simulink model "c00001M_harness"  (R2018a)
settings: Solver=FixedStepAuto  StartTime=0.0  StopTime=300  FixedStep=0.1  RelTol=1e-3
undefined symbols (not defined in the file): A1, hmax, R1, R2, sigbuilder_block, TempThreshold
(part 1 of 7)
settings Model: Creator=aarrieta  LastModifiedBy=umarkiegi

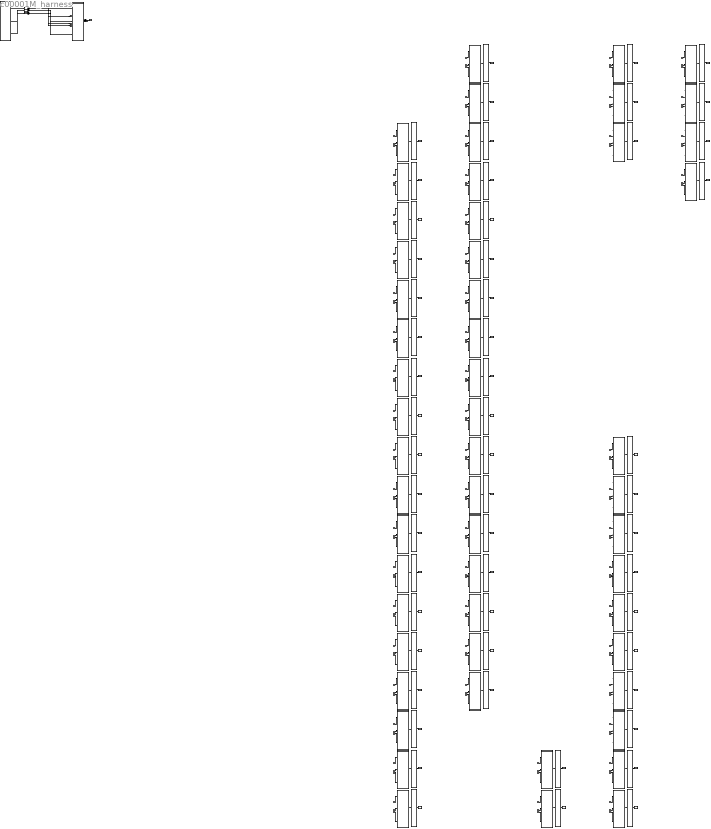
== system c00001M_harness ==
  CPSUT : Subsystem
  Eval100 : Subsystem
  Eval101 : Subsystem
  Eval102 : Subsystem
  Eval103 : Subsystem
  Eval104 : Subsystem
  Eval105 : Subsystem
  Eval106 : Subsystem
  Eval107 : Subsystem
  Eval108 : Subsystem
  Eval109 : Subsystem
  Eval110 : Subsystem
  Eval111 : Subsystem
  Eval112 : Subsystem
  Eval113 : Subsystem
  Eval114 : Subsystem
  Eval115 : Subsystem
  Eval116 : Subsystem
  Eval138 : Subsystem
  Eval139 : Subsystem
  Eval140 : Subsystem
  Eval141 : Subsystem
  Eval142 : Subsystem
  Eval150 : Subsystem
  Eval151 : Subsystem
  Eval152 : Subsystem
  Eval153 : Subsystem
  Eval154 : Subsystem
  Eval155 : Subsystem
  Eval156 : Subsystem
  Eval157 : Subsystem
  Eval158 : Subsystem
  Eval159 : Subsystem
  Eval160 : Subsystem
  Eval161 : Subsystem
  Eval162 : Subsystem
  Eval163 : Subsystem
  Eval82 : Subsystem
  Eval83 : Subsystem
  Eval84 : Subsystem
  Eval85 : Subsystem
  Eval86 : Subsystem
  Eval87 : Subsystem
  Eval88 : Subsystem
  Eval89 : Subsystem
  Eval90 : Subsystem
  Eval91 : Subsystem
  Eval92 : Subsystem
  Eval93 : Subsystem
  Eval94 : Subsystem
  Eval95 : Subsystem
  Eval96 : Subsystem
  Eval97 : Subsystem
  Eval98 : Subsystem
  Eval99 : Subsystem
  Inputs : Subsystem  Tag=STV Subsys  LoadFcn=sigbuilder_block('load');  StartFcn=sigbuilder_block('start');  StopFcn=sigbuilder_block('stop');  ClipboardFcn=sigbuilder_block('clipboard');  mask(Sigbuilder block){tuvar=[0:10]}
      mask init:
      | if ~strcmp(get_param(bdroot(gcb),'SimulationStatus'),'stopped'),tuvar = sigbuilder_block('maskInit'); end
      settings: CopyFcn=sigbuilder_block('copy');  DeleteFcn=sigbuilder_block('delete');  ModelCloseFcn=sigbuilder_block('modelClose');  PreSaveFcn=sigbuilder_block('preSave');  PauseFcn=sigbuilder_block('pause');  ContinueFcn=sigbuilder_block('continue');  NameChangeFcn=sigbuilder_block('namechange');  OpenFcn=sigbuilder_block('open',[276.75 163.5 675.75 486.75 ]);  CloseFcn=sigbuilder_block('close');
      mask Display: plot(0, 0, 100, 100,[2, 2, 32, 32, 2], [68, 8, 8, 68, 68],[32, 2], [38, 38], [32, 19, 2],[53, 60, 44], [32, 17, 17, 2],[16, 16, 31, 31]);txt = getActiveGroup(gcbh);text(2, 100, txt,'verticalAlignment', 'top');
  M083 : Subsystem
  M084 : Subsystem
  M085 : Subsystem
  M086 : Subsystem
  M087 : Subsystem
  M088 : Subsystem
  M089 : Subsystem
  M090 : Subsystem
  M091 : Subsystem
  M092 : Subsystem
  M093 : Subsystem
  M094 : Subsystem
  M095 : Subsystem
  M096 : Subsystem
  M097 : Subsystem
  M098 : Subsystem
  M099 : Subsystem
  M100 : Subsystem
  M101 : Subsystem
  M102 : Subsystem
  M103 : Subsystem
  M104 : Subsystem
  M105 : Subsystem
  M106 : Subsystem
  M107 : Subsystem
  M108 : Subsystem
  M109 : Subsystem
  M110 : Subsystem
  M111 : Subsystem
  M112 : Subsystem
  M113 : Subsystem
  M114 : Subsystem
  M115 : Subsystem
  M116 : Subsystem
  M117 : Subsystem
  M139 : Subsystem
  M140 : Subsystem
  M141 : Subsystem
  M142 : Subsystem
  M143 : Subsystem
  M151 : Subsystem
  M152 : Subsystem
  M153 : Subsystem
  M154 : Subsystem
  M155 : Subsystem
  M156 : Subsystem
  M157 : Subsystem
  M158 : Subsystem
  M159 : Subsystem
  M160 : Subsystem
  M161 : Subsystem
  M162 : Subsystem
  M163 : Subsystem
  M164 : Subsystem
  To Workspace100 : ToWorkspace  VariableName=mutant101  SampleTime=-1
  To Workspace101 : ToWorkspace  VariableName=mutant102  SampleTime=-1
  To Workspace102 : ToWorkspace  VariableName=mutant103  SampleTime=-1
  To Workspace103 : ToWorkspace  VariableName=mutant104  SampleTime=-1
  To Workspace104 : ToWorkspace  VariableName=mutant105  SampleTime=-1
  To Workspace105 : ToWorkspace  VariableName=mutant106  SampleTime=-1
  To Workspace106 : ToWorkspace  VariableName=mutant107  SampleTime=-1
  To Workspace107 : ToWorkspace  VariableName=mutant108  SampleTime=-1
  To Workspace108 : ToWorkspace  VariableName=mutant109  SampleTime=-1
  To Workspace109 : ToWorkspace  VariableName=mutant110  SampleTime=-1
  To Workspace110 : ToWorkspace  VariableName=mutant111  SampleTime=-1
  To Workspace111 : ToWorkspace  VariableName=mutant112  SampleTime=-1
  To Workspace112 : ToWorkspace  VariableName=mutant113  SampleTime=-1
  To Workspace113 : ToWorkspace  VariableName=mutant114  SampleTime=-1
  To Workspace114 : ToWorkspace  VariableName=mutant115  SampleTime=-1
  To Workspace115 : ToWorkspace  VariableName=mutant116  SampleTime=-1
  To Workspace116 : ToWorkspace  VariableName=mutant117  SampleTime=-1
  To Workspace138 : ToWorkspace  VariableName=mutant139  SampleTime=-1
  To Workspace139 : ToWorkspace  VariableName=mutant140  SampleTime=-1
  To Workspace140 : ToWorkspace  VariableName=mutant141  SampleTime=-1
  To Workspace141 : ToWorkspace  VariableName=mutant142  SampleTime=-1
  To Workspace142 : ToWorkspace  VariableName=mutant143  SampleTime=-1
  To Workspace150 : ToWorkspace  VariableName=mutant151  SampleTime=-1
  To Workspace151 : ToWorkspace  VariableName=mutant152  SampleTime=-1
  To Workspace152 : ToWorkspace  VariableName=mutant153  SampleTime=-1
  To Workspace153 : ToWorkspace  VariableName=mutant154  SampleTime=-1
  To Workspace154 : ToWorkspace  VariableName=mutant155  SampleTime=-1
  To Workspace155 : ToWorkspace  VariableName=mutant156  SampleTime=-1
  To Workspace156 : ToWorkspace  VariableName=mutant157  SampleTime=-1
  To Workspace157 : ToWorkspace  VariableName=mutant158  SampleTime=-1
  To Workspace158 : ToWorkspace  VariableName=mutant159  SampleTime=-1
  To Workspace159 : ToWorkspace  VariableName=mutant160  SampleTime=-1
  To Workspace160 : ToWorkspace  VariableName=mutant161  SampleTime=-1
  To Workspace161 : ToWorkspace  VariableName=mutant162  SampleTime=-1
  To Workspace162 : ToWorkspace  VariableName=mutant163  SampleTime=-1
  To Workspace163 : ToWorkspace  VariableName=mutant164  SampleTime=-1
  To Workspace82 : ToWorkspace  VariableName=mutant083  SampleTime=-1
  To Workspace83 : ToWorkspace  VariableName=mutant084  SampleTime=-1
  To Workspace84 : ToWorkspace  VariableName=mutant085  SampleTime=-1
  To Workspace85 : ToWorkspace  VariableName=mutant086  SampleTime=-1
  To Workspace86 : ToWorkspace  VariableName=mutant087  SampleTime=-1
  To Workspace87 : ToWorkspace  VariableName=mutant088  SampleTime=-1
  To Workspace88 : ToWorkspace  VariableName=mutant089  SampleTime=-1
  To Workspace89 : ToWorkspace  VariableName=mutant090  SampleTime=-1
  To Workspace90 : ToWorkspace  VariableName=mutant091  SampleTime=-1
  To Workspace91 : ToWorkspace  VariableName=mutant092  SampleTime=-1
  To Workspace92 : ToWorkspace  VariableName=mutant093  SampleTime=-1
  To Workspace93 : ToWorkspace  VariableName=mutant094  SampleTime=-1
  To Workspace94 : ToWorkspace  VariableName=mutant095  SampleTime=-1
  To Workspace95 : ToWorkspace  VariableName=mutant096  SampleTime=-1
  To Workspace96 : ToWorkspace  VariableName=mutant097  SampleTime=-1
  To Workspace97 : ToWorkspace  VariableName=mutant098  SampleTime=-1
  To Workspace98 : ToWorkspace  VariableName=mutant099  SampleTime=-1
  To Workspace99 : ToWorkspace  VariableName=mutant100  SampleTime=-1
  dtc_CT2 : DataTypeConversion
  dtc_EB2 : DataTypeConversion
  dtc_T2 : DataTypeConversion
  LL2 : Outport
  tag scope: out2=global
  wires:
  CPSUT/1(LL2) -> [out2], LL2/1
  [in7] -> M083/1(CT2)
  [in11] -> M083/2(T2)
  [in12] -> M083/3(EB2)
  M083/1(LL2) -> Eval82/1(In2)
  Eval82/1(Out1) -> To Workspace82/1
  [in7] -> M084/1(CT2)
  [in11] -> M084/2(T2)
  [in12] -> M084/3(EB2)
  M084/1(LL2) -> Eval83/1(In2)
  Eval83/1(Out1) -> To Workspace83/1
  [in7] -> M085/1(CT2)
  [in11] -> M085/2(T2)
  [in12] -> M085/3(EB2)
  M085/1(LL2) -> Eval84/1(In2)
  Eval84/1(Out1) -> To Workspace84/1
  [in7] -> M086/1(CT2)
  [in11] -> M086/2(T2)
  [in12] -> M086/3(EB2)
  M086/1(LL2) -> Eval85/1(In2)
  Eval85/1(Out1) -> To Workspace85/1
  [in7] -> M087/1(CT2)
  [in11] -> M087/2(T2)
  [in12] -> M087/3(EB2)
  M087/1(LL2) -> Eval86/1(In2)
  Eval86/1(Out1) -> To Workspace86/1
  [in7] -> M088/1(CT2)
  [in11] -> M088/2(T2)
  [in12] -> M088/3(EB2)
  M088/1(LL2) -> Eval87/1(In2)
  Eval87/1(Out1) -> To Workspace87/1
  [in7] -> M089/1(CT2)
  [in11] -> M089/2(T2)
  [in12] -> M089/3(EB2)
  M089/1(LL2) -> Eval88/1(In2)
  Eval88/1(Out1) -> To Workspace88/1
  [in7] -> M090/1(CT2)
  [in11] -> M090/2(T2)
  [in12] -> M090/3(EB2)
  M090/1(LL2) -> Eval89/1(In2)
  Eval89/1(Out1) -> To Workspace89/1
  [in7] -> M091/1(CT2)
  [in11] -> M091/2(T2)
  [in12] -> M091/3(EB2)
  M091/1(LL2) -> Eval90/1(In2)
  Eval90/1(Out1) -> To Workspace90/1
  [in7] -> M092/1(CT2)
  [in11] -> M092/2(T2)
  [in12] -> M092/3(EB2)
  M092/1(LL2) -> Eval91/1(In2)
  Eval91/1(Out1) -> To Workspace91/1
  [in7] -> M093/1(CT2)
  [in11] -> M093/2(T2)
  [in12] -> M093/3(EB2)
  M093/1(LL2) -> Eval92/1(In2)
  Eval92/1(Out1) -> To Workspace92/1
  [in7] -> M094/1(CT2)
  [in11] -> M094/2(T2)
  [in12] -> M094/3(EB2)
  M094/1(LL2) -> Eval93/1(In2)
  Eval93/1(Out1) -> To Workspace93/1
  [in7] -> M095/1(CT2)
  [in11] -> M095/2(T2)
  [in12] -> M095/3(EB2)
  M095/1(LL2) -> Eval94/1(In2)
  Eval94/1(Out1) -> To Workspace94/1
  [in7] -> M096/1(CT2)
  [in11] -> M096/2(T2)
  [in12] -> M096/3(EB2)
  M096/1(LL2) -> Eval95/1(In2)
  Eval95/1(Out1) -> To Workspace95/1
  [in7] -> M097/1(CT2)
  [in11] -> M097/2(T2)
  [in12] -> M097/3(EB2)
  M097/1(LL2) -> Eval96/1(In2)
  Eval96/1(Out1) -> To Workspace96/1
  [in7] -> M098/1(CT2)
  [in11] -> M098/2(T2)
  [in12] -> M098/3(EB2)
  M098/1(LL2) -> Eval97/1(In2)
  Eval97/1(Out1) -> To Workspace97/1
  [in7] -> M099/1(CT2)
  [in11] -> M099/2(T2)
  [in12] -> M099/3(EB2)
  M099/1(LL2) -> Eval98/1(In2)
  Eval98/1(Out1) -> To Workspace98/1
  [in7] -> M100/1(CT2)
  [in11] -> M100/2(T2)
  [in12] -> M100/3(EB2)
  M100/1(LL2) -> Eval99/1(In2)
  Eval99/1(Out1) -> To Workspace99/1
  [in7] -> M101/1(CT2)
  [in11] -> M101/2(T2)
  [in12] -> M101/3(EB2)
  M101/1(LL2) -> Eval100/1(In2)
  Eval100/1(Out1) -> To Workspace100/1
  [in7] -> M102/1(CT2)
  [in11] -> M102/2(T2)
  [in12] -> M102/3(EB2)
  M102/1(LL2) -> Eval101/1(In2)
  Eval101/1(Out1) -> To Workspace101/1
  [in7] -> M103/1(CT2)
  [in11] -> M103/2(T2)
  [in12] -> M103/3(EB2)
  M103/1(LL2) -> Eval102/1(In2)
  Eval102/1(Out1) -> To Workspace102/1
  [in7] -> M104/1(CT2)
  [in11] -> M104/2(T2)
  [in12] -> M104/3(EB2)
  M104/1(LL2) -> Eval103/1(In2)
  Eval103/1(Out1) -> To Workspace103/1
  [in7] -> M105/1(CT2)
  [in11] -> M105/2(T2)
  [in12] -> M105/3(EB2)
  M105/1(LL2) -> Eval104/1(In2)
  Eval104/1(Out1) -> To Workspace104/1
  [in7] -> M106/1(CT2)
  [in11] -> M106/2(T2)
  [in12] -> M106/3(EB2)
  M106/1(LL2) -> Eval105/1(In2)
  Eval105/1(Out1) -> To Workspace105/1
  [in7] -> M107/1(CT2)
  [in11] -> M107/2(T2)
  [in12] -> M107/3(EB2)
  M107/1(LL2) -> Eval106/1(In2)
  Eval106/1(Out1) -> To Workspace106/1
  [in7] -> M108/1(CT2)
  [in11] -> M108/2(T2)
  [in12] -> M108/3(EB2)
  M108/1(LL2) -> Eval107/1(In2)
  Eval107/1(Out1) -> To Workspace107/1
  [in7] -> M109/1(CT2)
  [in11] -> M109/2(T2)
  [in12] -> M109/3(EB2)
  M109/1(LL2) -> Eval108/1(In2)
  Eval108/1(Out1) -> To Workspace108/1
  [in7] -> M110/1(CT2)
  [in11] -> M110/2(T2)
  [in12] -> M110/3(EB2)
  M110/1(LL2) -> Eval109/1(In2)
  Eval109/1(Out1) -> To Workspace109/1
  [in7] -> M111/1(CT2)
  [in11] -> M111/2(T2)
  [in12] -> M111/3(EB2)
  M111/1(LL2) -> Eval110/1(In2)
  Eval110/1(Out1) -> To Workspace110/1
  [in7] -> M112/1(CT2)
  [in11] -> M112/2(T2)
  [in12] -> M112/3(EB2)
  M112/1(LL2) -> Eval111/1(In2)
  Eval111/1(Out1) -> To Workspace111/1
  [in7] -> M113/1(CT2)
  [in11] -> M113/2(T2)
  [in12] -> M113/3(EB2)
  M113/1(LL2) -> Eval112/1(In2)
  Eval112/1(Out1) -> To Workspace112/1
  [in7] -> M114/1(CT2)
  [in11] -> M114/2(T2)
  [in12] -> M114/3(EB2)
  M114/1(LL2) -> Eval113/1(In2)
  Eval113/1(Out1) -> To Workspace113/1
  [in7] -> M115/1(CT2)
  [in11] -> M115/2(T2)
  [in12] -> M115/3(EB2)
  M115/1(LL2) -> Eval114/1(In2)
  Eval114/1(Out1) -> To Workspace114/1
  [in7] -> M116/1(CT2)
  [in11] -> M116/2(T2)
  [in12] -> M116/3(EB2)
  M116/1(LL2) -> Eval115/1(In2)
  Eval115/1(Out1) -> To Workspace115/1
  [in7] -> M117/1(CT2)
  [in11] -> M117/2(T2)
  [in12] -> M117/3(EB2)
  M117/1(LL2) -> Eval116/1(In2)
  Eval116/1(Out1) -> To Workspace116/1
  [in7] -> M139/1(CT2)
  [in11] -> M139/2(T2)
  [in12] -> M139/3(EB2)
  M139/1(LL2) -> Eval138/1(In2)
  Eval138/1(Out1) -> To Workspace138/1
  [in7] -> M140/1(CT2)
  [in11] -> M140/2(T2)
  [in12] -> M140/3(EB2)
  M140/1(LL2) -> Eval139/1(In2)
  Eval139/1(Out1) -> To Workspace139/1
  [in7] -> M141/1(CT2)
  [in11] -> M141/2(T2)
  [in12] -> M141/3(EB2)
  M141/1(LL2) -> Eval140/1(In2)
  Eval140/1(Out1) -> To Workspace140/1
  [in7] -> M142/1(CT2)
  [in11] -> M142/2(T2)
  [in12] -> M142/3(EB2)
  M142/1(LL2) -> Eval141/1(In2)
  Eval141/1(Out1) -> To Workspace141/1
  [in7] -> M143/1(CT2)
  [in11] -> M143/2(T2)
  [in12] -> M143/3(EB2)
  M143/1(LL2) -> Eval142/1(In2)
  Eval142/1(Out1) -> To Workspace142/1
  [in7] -> M151/1(CT2)
  [in11] -> M151/2(T2)
  [in12] -> M151/3(EB2)
  M151/1(LL2) -> Eval150/1(In2)
  Eval150/1(Out1) -> To Workspace150/1
  [in7] -> M152/1(CT2)
  [in11] -> M152/2(T2)
  [in12] -> M152/3(EB2)
  M152/1(LL2) -> Eval151/1(In2)
  Eval151/1(Out1) -> To Workspace151/1
  [in7] -> M153/1(CT2)
  [in11] -> M153/2(T2)
  [in12] -> M153/3(EB2)
  M153/1(LL2) -> Eval152/1(In2)
  Eval152/1(Out1) -> To Workspace152/1
  [in7] -> M154/1(CT2)
  [in11] -> M154/2(T2)
  [in12] -> M154/3(EB2)
  M154/1(LL2) -> Eval153/1(In2)
  Eval153/1(Out1) -> To Workspace153/1
  [in7] -> M155/1(CT2)
  [in11] -> M155/2(T2)
  [in12] -> M155/3(EB2)
  M155/1(LL2) -> Eval154/1(In2)
  Eval154/1(Out1) -> To Workspace154/1
  [in7] -> M156/1(CT2)
  [in11] -> M156/2(T2)
  [in12] -> M156/3(EB2)
  M156/1(LL2) -> Eval155/1(In2)
  Eval155/1(Out1) -> To Workspace155/1
  [in7] -> M157/1(CT2)
  [in11] -> M157/2(T2)
  [in12] -> M157/3(EB2)
  M157/1(LL2) -> Eval156/1(In2)
  Eval156/1(Out1) -> To Workspace156/1
  [in7] -> M158/1(CT2)
  [in11] -> M158/2(T2)
  [in12] -> M158/3(EB2)
  M158/1(LL2) -> Eval157/1(In2)
  Eval157/1(Out1) -> To Workspace157/1
  [in7] -> M159/1(CT2)
  [in11] -> M159/2(T2)
  [in12] -> M159/3(EB2)
  M159/1(LL2) -> Eval158/1(In2)
  Eval158/1(Out1) -> To Workspace158/1
  [in7] -> M160/1(CT2)
  [in11] -> M160/2(T2)
  [in12] -> M160/3(EB2)
  M160/1(LL2) -> Eval159/1(In2)
  Eval159/1(Out1) -> To Workspace159/1
  [in7] -> M161/1(CT2)
  [in11] -> M161/2(T2)
  [in12] -> M161/3(EB2)
  M161/1(LL2) -> Eval160/1(In2)
  Eval160/1(Out1) -> To Workspace160/1
  [in7] -> M162/1(CT2)
  [in11] -> M162/2(T2)
  [in12] -> M162/3(EB2)
  M162/1(LL2) -> Eval161/1(In2)
  Eval161/1(Out1) -> To Workspace161/1
  [in7] -> M163/1(CT2)
  [in11] -> M163/2(T2)
  [in12] -> M163/3(EB2)
  M163/1(LL2) -> Eval162/1(In2)
  Eval162/1(Out1) -> To Workspace162/1
  [in7] -> M164/1(CT2)
  [in11] -> M164/2(T2)
  [in12] -> M164/3(EB2)
  M164/1(LL2) -> Eval163/1(In2)
  Eval163/1(Out1) -> To Workspace163/1
  Inputs/1(CT2) -> dtc_CT2/1
  dtc_CT2/1 -> CPSUT/1(CT2), [in7]
  Inputs/2(T2) -> dtc_T2/1
  dtc_T2/1 -> CPSUT/2(T2), [in11]
  Inputs/3(EB2) -> dtc_EB2/1
  dtc_EB2/1 -> CPSUT/3(EB2), [in12]

== system c00001M_harness/CPSUT ==
  note: VALUES
      | ---------------------------------
      | ControlType = 1 | 2 | 3
      | FillTank = 0 | 1
      | EmptyTank = 0 | 1
      | ManualReference between 0 and 1
      | Tempreature between 0 and 100
      | EmergencyButton = 0 | 1
      | LiquidLevel between 0 and 1 (hmax)
  note: Inputs For Tank2
  note: NAMES
      | --------------------------------------------
      | CT1 = ControlType Tank 1
      | F1 = Fill Tank 1
      | E1 = Empty Tank 1
      | MR1 = Manual Reference Tank1
      | T1 = Temperature Tank 1
      | EB1 = Emergency Button Tank 1
      | LL1 = Liquid Level 1
  note: Inputs For Tank3
  note: Inputs For Tank1
  CT2 : Inport
  T2 : Inport  Port=2
  EB2 : Inport  Port=3
  Tank2 : Subsystem
  LL2 : Outport
  wires:
  Tank2/1(LL2) -> LL2/1
  EB2/1 -> Tank2/3(EB2)
  CT2/1 -> Tank2/1(CT2)
  T2/1 -> Tank2/2(T2)

== system c00001M_harness/Eval100 ==
  In2 : Inport
  Constant1 : Constant
  Constant3 : Constant
  Data Type Conversion1 : DataTypeConversion
  Memory2 : Memory  InitialCondition=1
  MinMax : MinMax  Inputs=3
  MinMax2 : MinMax  Inputs=2
  ROOut2 : RelationalOperator  Operator===  OutDataTypeStr=boolean  RndMeth=Simplest
  Out1 : Outport
  wires:
  Data Type Conversion1/1 -> MinMax2/1
  MinMax2/1 -> MinMax/2, Memory2/1
  Memory2/1 -> MinMax2/2
  ROOut2/1 -> Data Type Conversion1/1
  [out2] -> ROOut2/2
  In2/1 -> ROOut2/1
  MinMax/1 -> Out1/1
  Constant1/1 -> MinMax/1
  Constant3/1 -> MinMax/3

== system c00001M_harness/Eval101 ==
  In2 : Inport
  Constant1 : Constant
  Constant3 : Constant
  Data Type Conversion1 : DataTypeConversion
  Memory2 : Memory  InitialCondition=1
  MinMax : MinMax  Inputs=3
  MinMax2 : MinMax  Inputs=2
  ROOut2 : RelationalOperator  Operator===  OutDataTypeStr=boolean  RndMeth=Simplest
  Out1 : Outport
  wires:
  Data Type Conversion1/1 -> MinMax2/1
  MinMax2/1 -> MinMax/2, Memory2/1
  Memory2/1 -> MinMax2/2
  ROOut2/1 -> Data Type Conversion1/1
  [out2] -> ROOut2/2
  In2/1 -> ROOut2/1
  MinMax/1 -> Out1/1
  Constant1/1 -> MinMax/1
  Constant3/1 -> MinMax/3

== system c00001M_harness/Eval102 ==
  In2 : Inport
  Constant1 : Constant
  Constant3 : Constant
  Data Type Conversion1 : DataTypeConversion
  Memory2 : Memory  InitialCondition=1
  MinMax : MinMax  Inputs=3
  MinMax2 : MinMax  Inputs=2
  ROOut2 : RelationalOperator  Operator===  OutDataTypeStr=boolean  RndMeth=Simplest
  Out1 : Outport
  wires:
  Data Type Conversion1/1 -> MinMax2/1
  MinMax2/1 -> MinMax/2, Memory2/1
  Memory2/1 -> MinMax2/2
  ROOut2/1 -> Data Type Conversion1/1
  [out2] -> ROOut2/2
  In2/1 -> ROOut2/1
  MinMax/1 -> Out1/1
  Constant1/1 -> MinMax/1
  Constant3/1 -> MinMax/3

== system c00001M_harness/Eval103 ==
  In2 : Inport
  Constant1 : Constant
  Constant3 : Constant
  Data Type Conversion1 : DataTypeConversion
  Memory2 : Memory  InitialCondition=1
  MinMax : MinMax  Inputs=3
  MinMax2 : MinMax  Inputs=2
  ROOut2 : RelationalOperator  Operator===  OutDataTypeStr=boolean  RndMeth=Simplest
  Out1 : Outport
  wires:
  Data Type Conversion1/1 -> MinMax2/1
  MinMax2/1 -> MinMax/2, Memory2/1
  Memory2/1 -> MinMax2/2
  ROOut2/1 -> Data Type Conversion1/1
  [out2] -> ROOut2/2
  In2/1 -> ROOut2/1
  MinMax/1 -> Out1/1
  Constant1/1 -> MinMax/1
  Constant3/1 -> MinMax/3

== system c00001M_harness/Eval104 ==
  In2 : Inport
  Constant1 : Constant
  Constant3 : Constant
  Data Type Conversion1 : DataTypeConversion
  Memory2 : Memory  InitialCondition=1
  MinMax : MinMax  Inputs=3
  MinMax2 : MinMax  Inputs=2
  ROOut2 : RelationalOperator  Operator===  OutDataTypeStr=boolean  RndMeth=Simplest
  Out1 : Outport
  wires:
  Data Type Conversion1/1 -> MinMax2/1
  MinMax2/1 -> MinMax/2, Memory2/1
  Memory2/1 -> MinMax2/2
  ROOut2/1 -> Data Type Conversion1/1
  [out2] -> ROOut2/2
  In2/1 -> ROOut2/1
  MinMax/1 -> Out1/1
  Constant1/1 -> MinMax/1
  Constant3/1 -> MinMax/3

== system c00001M_harness/Eval105 ==
  In2 : Inport
  Constant1 : Constant
  Constant3 : Constant
  Data Type Conversion1 : DataTypeConversion
  Memory2 : Memory  InitialCondition=1
  MinMax : MinMax  Inputs=3
  MinMax2 : MinMax  Inputs=2
  ROOut2 : RelationalOperator  Operator===  OutDataTypeStr=boolean  RndMeth=Simplest
  Out1 : Outport
  wires:
  Data Type Conversion1/1 -> MinMax2/1
  MinMax2/1 -> MinMax/2, Memory2/1
  Memory2/1 -> MinMax2/2
  ROOut2/1 -> Data Type Conversion1/1
  [out2] -> ROOut2/2
  In2/1 -> ROOut2/1
  MinMax/1 -> Out1/1
  Constant1/1 -> MinMax/1
  Constant3/1 -> MinMax/3

== system c00001M_harness/Eval106 ==
  In2 : Inport
  Constant1 : Constant
  Constant3 : Constant
  Data Type Conversion1 : DataTypeConversion
  Memory2 : Memory  InitialCondition=1
  MinMax : MinMax  Inputs=3
  MinMax2 : MinMax  Inputs=2
  ROOut2 : RelationalOperator  Operator===  OutDataTypeStr=boolean  RndMeth=Simplest
  Out1 : Outport
  wires:
  Data Type Conversion1/1 -> MinMax2/1
  MinMax2/1 -> MinMax/2, Memory2/1
  Memory2/1 -> MinMax2/2
  ROOut2/1 -> Data Type Conversion1/1
  [out2] -> ROOut2/2
  In2/1 -> ROOut2/1
  MinMax/1 -> Out1/1
  Constant1/1 -> MinMax/1
  Constant3/1 -> MinMax/3

== system c00001M_harness/Eval107 ==
  In2 : Inport
  Constant1 : Constant
  Constant3 : Constant
  Data Type Conversion1 : DataTypeConversion
  Memory2 : Memory  InitialCondition=1
  MinMax : MinMax  Inputs=3
  MinMax2 : MinMax  Inputs=2
  ROOut2 : RelationalOperator  Operator===  OutDataTypeStr=boolean  RndMeth=Simplest
  Out1 : Outport
  wires:
  Data Type Conversion1/1 -> MinMax2/1
  MinMax2/1 -> MinMax/2, Memory2/1
  Memory2/1 -> MinMax2/2
  ROOut2/1 -> Data Type Conversion1/1
  [out2] -> ROOut2/2
  In2/1 -> ROOut2/1
  MinMax/1 -> Out1/1
  Constant1/1 -> MinMax/1
  Constant3/1 -> MinMax/3

== system c00001M_harness/Eval108 ==
  In2 : Inport
  Constant1 : Constant
  Constant3 : Constant
  Data Type Conversion1 : DataTypeConversion
  Memory2 : Memory  InitialCondition=1
  MinMax : MinMax  Inputs=3
  MinMax2 : MinMax  Inputs=2
  ROOut2 : RelationalOperator  Operator===  OutDataTypeStr=boolean  RndMeth=Simplest
  Out1 : Outport
  wires:
  Data Type Conversion1/1 -> MinMax2/1
  MinMax2/1 -> MinMax/2, Memory2/1
  Memory2/1 -> MinMax2/2
  ROOut2/1 -> Data Type Conversion1/1
  [out2] -> ROOut2/2
  In2/1 -> ROOut2/1
  MinMax/1 -> Out1/1
  Constant1/1 -> MinMax/1
  Constant3/1 -> MinMax/3

== system c00001M_harness/Eval109 ==
  In2 : Inport
  Constant1 : Constant
  Constant3 : Constant
  Data Type Conversion1 : DataTypeConversion
  Memory2 : Memory  InitialCondition=1
  MinMax : MinMax  Inputs=3
  MinMax2 : MinMax  Inputs=2
  ROOut2 : RelationalOperator  Operator===  OutDataTypeStr=boolean  RndMeth=Simplest
  Out1 : Outport
  wires:
  Data Type Conversion1/1 -> MinMax2/1
  MinMax2/1 -> MinMax/2, Memory2/1
  Memory2/1 -> MinMax2/2
  ROOut2/1 -> Data Type Conversion1/1
  [out2] -> ROOut2/2
  In2/1 -> ROOut2/1
  MinMax/1 -> Out1/1
  Constant1/1 -> MinMax/1
  Constant3/1 -> MinMax/3

== system c00001M_harness/Eval110 ==
  In2 : Inport
  Constant1 : Constant
  Constant3 : Constant
  Data Type Conversion1 : DataTypeConversion
  Memory2 : Memory  InitialCondition=1
  MinMax : MinMax  Inputs=3
  MinMax2 : MinMax  Inputs=2
  ROOut2 : RelationalOperator  Operator===  OutDataTypeStr=boolean  RndMeth=Simplest
  Out1 : Outport
  wires:
  Data Type Conversion1/1 -> MinMax2/1
  MinMax2/1 -> MinMax/2, Memory2/1
  Memory2/1 -> MinMax2/2
  ROOut2/1 -> Data Type Conversion1/1
  [out2] -> ROOut2/2
  In2/1 -> ROOut2/1
  MinMax/1 -> Out1/1
  Constant1/1 -> MinMax/1
  Constant3/1 -> MinMax/3

== system c00001M_harness/Eval111 ==
  In2 : Inport
  Constant1 : Constant
  Constant3 : Constant
  Data Type Conversion1 : DataTypeConversion
  Memory2 : Memory  InitialCondition=1
  MinMax : MinMax  Inputs=3
  MinMax2 : MinMax  Inputs=2
  ROOut2 : RelationalOperator  Operator===  OutDataTypeStr=boolean  RndMeth=Simplest
  Out1 : Outport
  wires:
  Data Type Conversion1/1 -> MinMax2/1
  MinMax2/1 -> MinMax/2, Memory2/1
  Memory2/1 -> MinMax2/2
  ROOut2/1 -> Data Type Conversion1/1
  [out2] -> ROOut2/2
  In2/1 -> ROOut2/1
  MinMax/1 -> Out1/1
  Constant1/1 -> MinMax/1
  Constant3/1 -> MinMax/3

== system c00001M_harness/Eval112 ==
  In2 : Inport
  Constant1 : Constant
  Constant3 : Constant
  Data Type Conversion1 : DataTypeConversion
  Memory2 : Memory  InitialCondition=1
  MinMax : MinMax  Inputs=3
  MinMax2 : MinMax  Inputs=2
  ROOut2 : RelationalOperator  Operator===  OutDataTypeStr=boolean  RndMeth=Simplest
  Out1 : Outport
  wires:
  Data Type Conversion1/1 -> MinMax2/1
  MinMax2/1 -> MinMax/2, Memory2/1
  Memory2/1 -> MinMax2/2
  ROOut2/1 -> Data Type Conversion1/1
  [out2] -> ROOut2/2
  In2/1 -> ROOut2/1
  MinMax/1 -> Out1/1
  Constant1/1 -> MinMax/1
  Constant3/1 -> MinMax/3

== system c00001M_harness/Eval113 ==
  In2 : Inport
  Constant1 : Constant
  Constant3 : Constant
  Data Type Conversion1 : DataTypeConversion
  Memory2 : Memory  InitialCondition=1
  MinMax : MinMax  Inputs=3
  MinMax2 : MinMax  Inputs=2
  ROOut2 : RelationalOperator  Operator===  OutDataTypeStr=boolean  RndMeth=Simplest
  Out1 : Outport
  wires:
  Data Type Conversion1/1 -> MinMax2/1
  MinMax2/1 -> MinMax/2, Memory2/1
  Memory2/1 -> MinMax2/2
  ROOut2/1 -> Data Type Conversion1/1
  [out2] -> ROOut2/2
  In2/1 -> ROOut2/1
  MinMax/1 -> Out1/1
  Constant1/1 -> MinMax/1
  Constant3/1 -> MinMax/3

== system c00001M_harness/Eval114 ==
  In2 : Inport
  Constant1 : Constant
  Constant3 : Constant
  Data Type Conversion1 : DataTypeConversion
  Memory2 : Memory  InitialCondition=1
  MinMax : MinMax  Inputs=3
  MinMax2 : MinMax  Inputs=2
  ROOut2 : RelationalOperator  Operator===  OutDataTypeStr=boolean  RndMeth=Simplest
  Out1 : Outport
  wires:
  Data Type Conversion1/1 -> MinMax2/1
  MinMax2/1 -> MinMax/2, Memory2/1
  Memory2/1 -> MinMax2/2
  ROOut2/1 -> Data Type Conversion1/1
  [out2] -> ROOut2/2
  In2/1 -> ROOut2/1
  MinMax/1 -> Out1/1
  Constant1/1 -> MinMax/1
  Constant3/1 -> MinMax/3

== system c00001M_harness/Eval115 ==
  In2 : Inport
  Constant1 : Constant
  Constant3 : Constant
  Data Type Conversion1 : DataTypeConversion
  Memory2 : Memory  InitialCondition=1
  MinMax : MinMax  Inputs=3
  MinMax2 : MinMax  Inputs=2
  ROOut2 : RelationalOperator  Operator===  OutDataTypeStr=boolean  RndMeth=Simplest
  Out1 : Outport
  wires:
  Data Type Conversion1/1 -> MinMax2/1
  MinMax2/1 -> MinMax/2, Memory2/1
  Memory2/1 -> MinMax2/2
  ROOut2/1 -> Data Type Conversion1/1
  [out2] -> ROOut2/2
  In2/1 -> ROOut2/1
  MinMax/1 -> Out1/1
  Constant1/1 -> MinMax/1
  Constant3/1 -> MinMax/3

== system c00001M_harness/Eval116 ==
  In2 : Inport
  Constant1 : Constant
  Constant3 : Constant
  Data Type Conversion1 : DataTypeConversion
  Memory2 : Memory  InitialCondition=1
  MinMax : MinMax  Inputs=3
  MinMax2 : MinMax  Inputs=2
  ROOut2 : RelationalOperator  Operator===  OutDataTypeStr=boolean  RndMeth=Simplest
  Out1 : Outport
  wires:
  Data Type Conversion1/1 -> MinMax2/1
  MinMax2/1 -> MinMax/2, Memory2/1
  Memory2/1 -> MinMax2/2
  ROOut2/1 -> Data Type Conversion1/1
  [out2] -> ROOut2/2
  In2/1 -> ROOut2/1
  MinMax/1 -> Out1/1
  Constant1/1 -> MinMax/1
  Constant3/1 -> MinMax/3

== system c00001M_harness/Eval138 ==
  In2 : Inport
  Constant1 : Constant
  Constant3 : Constant
  Data Type Conversion1 : DataTypeConversion
  Memory2 : Memory  InitialCondition=1
  MinMax : MinMax  Inputs=3
  MinMax2 : MinMax  Inputs=2
  ROOut2 : RelationalOperator  Operator===  OutDataTypeStr=boolean  RndMeth=Simplest
  Out1 : Outport
  wires:
  Data Type Conversion1/1 -> MinMax2/1
  MinMax2/1 -> MinMax/2, Memory2/1
  Memory2/1 -> MinMax2/2
  ROOut2/1 -> Data Type Conversion1/1
  [out2] -> ROOut2/2
  In2/1 -> ROOut2/1
  MinMax/1 -> Out1/1
  Constant1/1 -> MinMax/1
  Constant3/1 -> MinMax/3

== system c00001M_harness/Eval139 ==
  In2 : Inport
  Constant1 : Constant
  Constant3 : Constant
  Data Type Conversion1 : DataTypeConversion
  Memory2 : Memory  InitialCondition=1
  MinMax : MinMax  Inputs=3
  MinMax2 : MinMax  Inputs=2
  ROOut2 : RelationalOperator  Operator===  OutDataTypeStr=boolean  RndMeth=Simplest
  Out1 : Outport
  wires:
  Data Type Conversion1/1 -> MinMax2/1
  MinMax2/1 -> MinMax/2, Memory2/1
  Memory2/1 -> MinMax2/2
  ROOut2/1 -> Data Type Conversion1/1
  [out2] -> ROOut2/2
  In2/1 -> ROOut2/1
  MinMax/1 -> Out1/1
  Constant1/1 -> MinMax/1
  Constant3/1 -> MinMax/3

== system c00001M_harness/Eval140 ==
  In2 : Inport
  Constant1 : Constant
  Constant3 : Constant
  Data Type Conversion1 : DataTypeConversion
  Memory2 : Memory  InitialCondition=1
  MinMax : MinMax  Inputs=3
  MinMax2 : MinMax  Inputs=2
  ROOut2 : RelationalOperator  Operator===  OutDataTypeStr=boolean  RndMeth=Simplest
  Out1 : Outport
  wires:
  Data Type Conversion1/1 -> MinMax2/1
  MinMax2/1 -> MinMax/2, Memory2/1
  Memory2/1 -> MinMax2/2
  ROOut2/1 -> Data Type Conversion1/1
  [out2] -> ROOut2/2
  In2/1 -> ROOut2/1
  MinMax/1 -> Out1/1
  Constant1/1 -> MinMax/1
  Constant3/1 -> MinMax/3

== system c00001M_harness/Eval141 ==
  In2 : Inport
  Constant1 : Constant
  Constant3 : Constant
  Data Type Conversion1 : DataTypeConversion
  Memory2 : Memory  InitialCondition=1
  MinMax : MinMax  Inputs=3
  MinMax2 : MinMax  Inputs=2
  ROOut2 : RelationalOperator  Operator===  OutDataTypeStr=boolean  RndMeth=Simplest
  Out1 : Outport
  wires:
  Data Type Conversion1/1 -> MinMax2/1
  MinMax2/1 -> MinMax/2, Memory2/1
  Memory2/1 -> MinMax2/2
  ROOut2/1 -> Data Type Conversion1/1
  [out2] -> ROOut2/2
  In2/1 -> ROOut2/1
  MinMax/1 -> Out1/1
  Constant1/1 -> MinMax/1
  Constant3/1 -> MinMax/3

== system c00001M_harness/Eval142 ==
  In2 : Inport
  Constant1 : Constant
  Constant3 : Constant
  Data Type Conversion1 : DataTypeConversion
  Memory2 : Memory  InitialCondition=1
  MinMax : MinMax  Inputs=3
  MinMax2 : MinMax  Inputs=2
  ROOut2 : RelationalOperator  Operator===  OutDataTypeStr=boolean  RndMeth=Simplest
  Out1 : Outport
  wires:
  Data Type Conversion1/1 -> MinMax2/1
  MinMax2/1 -> MinMax/2, Memory2/1
  Memory2/1 -> MinMax2/2
  ROOut2/1 -> Data Type Conversion1/1
  [out2] -> ROOut2/2
  In2/1 -> ROOut2/1
  MinMax/1 -> Out1/1
  Constant1/1 -> MinMax/1
  Constant3/1 -> MinMax/3

== system c00001M_harness/Eval150 ==
  In2 : Inport
  Constant1 : Constant
  Constant3 : Constant
  Data Type Conversion1 : DataTypeConversion
  Memory2 : Memory  InitialCondition=1
  MinMax : MinMax  Inputs=3
  MinMax2 : MinMax  Inputs=2
  ROOut2 : RelationalOperator  Operator===  OutDataTypeStr=boolean  RndMeth=Simplest
  Out1 : Outport
  wires:
  Data Type Conversion1/1 -> MinMax2/1
  MinMax2/1 -> MinMax/2, Memory2/1
  Memory2/1 -> MinMax2/2
  ROOut2/1 -> Data Type Conversion1/1
  [out2] -> ROOut2/2
  In2/1 -> ROOut2/1
  MinMax/1 -> Out1/1
  Constant1/1 -> MinMax/1
  Constant3/1 -> MinMax/3

== system c00001M_harness/Eval151 ==
  In2 : Inport
  Constant1 : Constant
  Constant3 : Constant
  Data Type Conversion1 : DataTypeConversion
  Memory2 : Memory  InitialCondition=1
  MinMax : MinMax  Inputs=3
  MinMax2 : MinMax  Inputs=2
  ROOut2 : RelationalOperator  Operator===  OutDataTypeStr=boolean  RndMeth=Simplest
  Out1 : Outport
  wires:
  Data Type Conversion1/1 -> MinMax2/1
  MinMax2/1 -> MinMax/2, Memory2/1
  Memory2/1 -> MinMax2/2
  ROOut2/1 -> Data Type Conversion1/1
  [out2] -> ROOut2/2
  In2/1 -> ROOut2/1
  MinMax/1 -> Out1/1
  Constant1/1 -> MinMax/1
  Constant3/1 -> MinMax/3

== system c00001M_harness/Eval152 ==
  In2 : Inport
  Constant1 : Constant
  Constant3 : Constant
  Data Type Conversion1 : DataTypeConversion
  Memory2 : Memory  InitialCondition=1
  MinMax : MinMax  Inputs=3
  MinMax2 : MinMax  Inputs=2
  ROOut2 : RelationalOperator  Operator===  OutDataTypeStr=boolean  RndMeth=Simplest
  Out1 : Outport
  wires:
  Data Type Conversion1/1 -> MinMax2/1
  MinMax2/1 -> MinMax/2, Memory2/1
  Memory2/1 -> MinMax2/2
  ROOut2/1 -> Data Type Conversion1/1
  [out2] -> ROOut2/2
  In2/1 -> ROOut2/1
  MinMax/1 -> Out1/1
  Constant1/1 -> MinMax/1
  Constant3/1 -> MinMax/3

== system c00001M_harness/Eval153 ==
  In2 : Inport
  Constant1 : Constant
  Constant3 : Constant
  Data Type Conversion1 : DataTypeConversion
  Memory2 : Memory  InitialCondition=1
  MinMax : MinMax  Inputs=3
  MinMax2 : MinMax  Inputs=2
  ROOut2 : RelationalOperator  Operator===  OutDataTypeStr=boolean  RndMeth=Simplest
  Out1 : Outport
  wires:
  Data Type Conversion1/1 -> MinMax2/1
  MinMax2/1 -> MinMax/2, Memory2/1
  Memory2/1 -> MinMax2/2
  ROOut2/1 -> Data Type Conversion1/1
  [out2] -> ROOut2/2
  In2/1 -> ROOut2/1
  MinMax/1 -> Out1/1
  Constant1/1 -> MinMax/1
  Constant3/1 -> MinMax/3

== system c00001M_harness/Eval154 ==
  In2 : Inport
  Constant1 : Constant
  Constant3 : Constant
  Data Type Conversion1 : DataTypeConversion
  Memory2 : Memory  InitialCondition=1
  MinMax : MinMax  Inputs=3
  MinMax2 : MinMax  Inputs=2
  ROOut2 : RelationalOperator  Operator===  OutDataTypeStr=boolean  RndMeth=Simplest
  Out1 : Outport
  wires:
  Data Type Conversion1/1 -> MinMax2/1
  MinMax2/1 -> MinMax/2, Memory2/1
  Memory2/1 -> MinMax2/2
  ROOut2/1 -> Data Type Conversion1/1
  [out2] -> ROOut2/2
  In2/1 -> ROOut2/1
  MinMax/1 -> Out1/1
  Constant1/1 -> MinMax/1
  Constant3/1 -> MinMax/3

== system c00001M_harness/Eval155 ==
  In2 : Inport
  Constant1 : Constant
  Constant3 : Constant
  Data Type Conversion1 : DataTypeConversion
  Memory2 : Memory  InitialCondition=1
  MinMax : MinMax  Inputs=3
  MinMax2 : MinMax  Inputs=2
  ROOut2 : RelationalOperator  Operator===  OutDataTypeStr=boolean  RndMeth=Simplest
  Out1 : Outport
  wires:
  Data Type Conversion1/1 -> MinMax2/1
  MinMax2/1 -> MinMax/2, Memory2/1
  Memory2/1 -> MinMax2/2
  ROOut2/1 -> Data Type Conversion1/1
  [out2] -> ROOut2/2
  In2/1 -> ROOut2/1
  MinMax/1 -> Out1/1
  Constant1/1 -> MinMax/1
  Constant3/1 -> MinMax/3

== system c00001M_harness/Eval156 ==
  In2 : Inport
  Constant1 : Constant
  Constant3 : Constant
  Data Type Conversion1 : DataTypeConversion
  Memory2 : Memory  InitialCondition=1
  MinMax : MinMax  Inputs=3
  MinMax2 : MinMax  Inputs=2
  ROOut2 : RelationalOperator  Operator===  OutDataTypeStr=boolean  RndMeth=Simplest
  Out1 : Outport
  wires:
  Data Type Conversion1/1 -> MinMax2/1
  MinMax2/1 -> MinMax/2, Memory2/1
  Memory2/1 -> MinMax2/2
  ROOut2/1 -> Data Type Conversion1/1
  [out2] -> ROOut2/2
  In2/1 -> ROOut2/1
  MinMax/1 -> Out1/1
  Constant1/1 -> MinMax/1
  Constant3/1 -> MinMax/3

== system c00001M_harness/Eval157 ==
  In2 : Inport
  Constant1 : Constant
  Constant3 : Constant
  Data Type Conversion1 : DataTypeConversion
  Memory2 : Memory  InitialCondition=1
  MinMax : MinMax  Inputs=3
  MinMax2 : MinMax  Inputs=2
  ROOut2 : RelationalOperator  Operator===  OutDataTypeStr=boolean  RndMeth=Simplest
  Out1 : Outport
  wires:
  Data Type Conversion1/1 -> MinMax2/1
  MinMax2/1 -> MinMax/2, Memory2/1
  Memory2/1 -> MinMax2/2
  ROOut2/1 -> Data Type Conversion1/1
  [out2] -> ROOut2/2
  In2/1 -> ROOut2/1
  MinMax/1 -> Out1/1
  Constant1/1 -> MinMax/1
  Constant3/1 -> MinMax/3

== system c00001M_harness/Eval158 ==
  In2 : Inport
  Constant1 : Constant
  Constant3 : Constant
  Data Type Conversion1 : DataTypeConversion
  Memory2 : Memory  InitialCondition=1
  MinMax : MinMax  Inputs=3
  MinMax2 : MinMax  Inputs=2
  ROOut2 : RelationalOperator  Operator===  OutDataTypeStr=boolean  RndMeth=Simplest
  Out1 : Outport
  wires:
  Data Type Conversion1/1 -> MinMax2/1
  MinMax2/1 -> MinMax/2, Memory2/1
  Memory2/1 -> MinMax2/2
  ROOut2/1 -> Data Type Conversion1/1
  [out2] -> ROOut2/2
  In2/1 -> ROOut2/1
  MinMax/1 -> Out1/1
  Constant1/1 -> MinMax/1
  Constant3/1 -> MinMax/3

== system c00001M_harness/Eval159 ==
  In2 : Inport
  Constant1 : Constant
  Constant3 : Constant
  Data Type Conversion1 : DataTypeConversion
  Memory2 : Memory  InitialCondition=1
  MinMax : MinMax  Inputs=3
  MinMax2 : MinMax  Inputs=2
  ROOut2 : RelationalOperator  Operator===  OutDataTypeStr=boolean  RndMeth=Simplest
  Out1 : Outport
  wires:
  Data Type Conversion1/1 -> MinMax2/1
  MinMax2/1 -> MinMax/2, Memory2/1
  Memory2/1 -> MinMax2/2
  ROOut2/1 -> Data Type Conversion1/1
  [out2] -> ROOut2/2
  In2/1 -> ROOut2/1
  MinMax/1 -> Out1/1
  Constant1/1 -> MinMax/1
  Constant3/1 -> MinMax/3

== system c00001M_harness/Eval160 ==
  In2 : Inport
  Constant1 : Constant
  Constant3 : Constant
  Data Type Conversion1 : DataTypeConversion
  Memory2 : Memory  InitialCondition=1
  MinMax : MinMax  Inputs=3
  MinMax2 : MinMax  Inputs=2
  ROOut2 : RelationalOperator  Operator===  OutDataTypeStr=boolean  RndMeth=Simplest
  Out1 : Outport
  wires:
  Data Type Conversion1/1 -> MinMax2/1
  MinMax2/1 -> MinMax/2, Memory2/1
  Memory2/1 -> MinMax2/2
  ROOut2/1 -> Data Type Conversion1/1
  [out2] -> ROOut2/2
  In2/1 -> ROOut2/1
  MinMax/1 -> Out1/1
  Constant1/1 -> MinMax/1
  Constant3/1 -> MinMax/3

== system c00001M_harness/Eval161 ==
  In2 : Inport
  Constant1 : Constant
  Constant3 : Constant
  Data Type Conversion1 : DataTypeConversion
  Memory2 : Memory  InitialCondition=1
  MinMax : MinMax  Inputs=3
  MinMax2 : MinMax  Inputs=2
  ROOut2 : RelationalOperator  Operator===  OutDataTypeStr=boolean  RndMeth=Simplest
  Out1 : Outport
  wires:
  Data Type Conversion1/1 -> MinMax2/1
  MinMax2/1 -> MinMax/2, Memory2/1
  Memory2/1 -> MinMax2/2
  ROOut2/1 -> Data Type Conversion1/1
  [out2] -> ROOut2/2
  In2/1 -> ROOut2/1
  MinMax/1 -> Out1/1
  Constant1/1 -> MinMax/1
  Constant3/1 -> MinMax/3

== system c00001M_harness/Eval162 ==
  In2 : Inport
  Constant1 : Constant
  Constant3 : Constant
  Data Type Conversion1 : DataTypeConversion
  Memory2 : Memory  InitialCondition=1
  MinMax : MinMax  Inputs=3
  MinMax2 : MinMax  Inputs=2
  ROOut2 : RelationalOperator  Operator===  OutDataTypeStr=boolean  RndMeth=Simplest
  Out1 : Outport
  wires:
  Data Type Conversion1/1 -> MinMax2/1
  MinMax2/1 -> MinMax/2, Memory2/1
  Memory2/1 -> MinMax2/2
  ROOut2/1 -> Data Type Conversion1/1
  [out2] -> ROOut2/2
  In2/1 -> ROOut2/1
  MinMax/1 -> Out1/1
  Constant1/1 -> MinMax/1
  Constant3/1 -> MinMax/3

== system c00001M_harness/Eval163 ==
  In2 : Inport
  Constant1 : Constant
  Constant3 : Constant
  Data Type Conversion1 : DataTypeConversion
  Memory2 : Memory  InitialCondition=1
  MinMax : MinMax  Inputs=3
  MinMax2 : MinMax  Inputs=2
  ROOut2 : RelationalOperator  Operator===  OutDataTypeStr=boolean  RndMeth=Simplest
  Out1 : Outport
  wires:
  Data Type Conversion1/1 -> MinMax2/1
  MinMax2/1 -> MinMax/2, Memory2/1
  Memory2/1 -> MinMax2/2
  ROOut2/1 -> Data Type Conversion1/1
  [out2] -> ROOut2/2
  In2/1 -> ROOut2/1
  MinMax/1 -> Out1/1
  Constant1/1 -> MinMax/1
  Constant3/1 -> MinMax/3

== system c00001M_harness/Eval82 ==
  In2 : Inport
  Constant1 : Constant
  Constant3 : Constant
  Data Type Conversion1 : DataTypeConversion
  Memory2 : Memory  InitialCondition=1
  MinMax : MinMax  Inputs=3
  MinMax2 : MinMax  Inputs=2
  ROOut2 : RelationalOperator  Operator===  OutDataTypeStr=boolean  RndMeth=Simplest
  Out1 : Outport
  wires:
  Data Type Conversion1/1 -> MinMax2/1
  MinMax2/1 -> MinMax/2, Memory2/1
  Memory2/1 -> MinMax2/2
  ROOut2/1 -> Data Type Conversion1/1
  [out2] -> ROOut2/2
  In2/1 -> ROOut2/1
  MinMax/1 -> Out1/1
  Constant1/1 -> MinMax/1
  Constant3/1 -> MinMax/3

== system c00001M_harness/Eval83 ==
  In2 : Inport
  Constant1 : Constant
  Constant3 : Constant
  Data Type Conversion1 : DataTypeConversion
  Memory2 : Memory  InitialCondition=1
  MinMax : MinMax  Inputs=3
  MinMax2 : MinMax  Inputs=2
  ROOut2 : RelationalOperator  Operator===  OutDataTypeStr=boolean  RndMeth=Simplest
  Out1 : Outport
  wires:
  Data Type Conversion1/1 -> MinMax2/1
  MinMax2/1 -> MinMax/2, Memory2/1
  Memory2/1 -> MinMax2/2
  ROOut2/1 -> Data Type Conversion1/1
  [out2] -> ROOut2/2
  In2/1 -> ROOut2/1
  MinMax/1 -> Out1/1
  Constant1/1 -> MinMax/1
  Constant3/1 -> MinMax/3

== system c00001M_harness/Eval84 ==
  In2 : Inport
  Constant1 : Constant
  Constant3 : Constant
  Data Type Conversion1 : DataTypeConversion
  Memory2 : Memory  InitialCondition=1
  MinMax : MinMax  Inputs=3
  MinMax2 : MinMax  Inputs=2
  ROOut2 : RelationalOperator  Operator===  OutDataTypeStr=boolean  RndMeth=Simplest
  Out1 : Outport
  wires:
  Data Type Conversion1/1 -> MinMax2/1
  MinMax2/1 -> MinMax/2, Memory2/1
  Memory2/1 -> MinMax2/2
  ROOut2/1 -> Data Type Conversion1/1
  [out2] -> ROOut2/2
  In2/1 -> ROOut2/1
  MinMax/1 -> Out1/1
  Constant1/1 -> MinMax/1
  Constant3/1 -> MinMax/3

== system c00001M_harness/Eval85 ==
  In2 : Inport
  Constant1 : Constant
  Constant3 : Constant
  Data Type Conversion1 : DataTypeConversion
  Memory2 : Memory  InitialCondition=1
  MinMax : MinMax  Inputs=3
  MinMax2 : MinMax  Inputs=2
  ROOut2 : RelationalOperator  Operator===  OutDataTypeStr=boolean  RndMeth=Simplest
  Out1 : Outport
  wires:
  Data Type Conversion1/1 -> MinMax2/1
  MinMax2/1 -> MinMax/2, Memory2/1
  Memory2/1 -> MinMax2/2
  ROOut2/1 -> Data Type Conversion1/1
  [out2] -> ROOut2/2
  In2/1 -> ROOut2/1
  MinMax/1 -> Out1/1
  Constant1/1 -> MinMax/1
  Constant3/1 -> MinMax/3

== system c00001M_harness/Eval86 ==
  In2 : Inport
  Constant1 : Constant
  Constant3 : Constant
  Data Type Conversion1 : DataTypeConversion
  Memory2 : Memory  InitialCondition=1
  MinMax : MinMax  Inputs=3
  MinMax2 : MinMax  Inputs=2
  ROOut2 : RelationalOperator  Operator===  OutDataTypeStr=boolean  RndMeth=Simplest
  Out1 : Outport
  wires:
  Data Type Conversion1/1 -> MinMax2/1
  MinMax2/1 -> MinMax/2, Memory2/1
  Memory2/1 -> MinMax2/2
  ROOut2/1 -> Data Type Conversion1/1
  [out2] -> ROOut2/2
  In2/1 -> ROOut2/1
  MinMax/1 -> Out1/1
  Constant1/1 -> MinMax/1
  Constant3/1 -> MinMax/3

== system c00001M_harness/Eval87 ==
  In2 : Inport
  Constant1 : Constant
  Constant3 : Constant
  Data Type Conversion1 : DataTypeConversion
  Memory2 : Memory  InitialCondition=1
  MinMax : MinMax  Inputs=3
  MinMax2 : MinMax  Inputs=2
  ROOut2 : RelationalOperator  Operator===  OutDataTypeStr=boolean  RndMeth=Simplest
  Out1 : Outport
  wires:
  Data Type Conversion1/1 -> MinMax2/1
  MinMax2/1 -> MinMax/2, Memory2/1
  Memory2/1 -> MinMax2/2
  ROOut2/1 -> Data Type Conversion1/1
  [out2] -> ROOut2/2
  In2/1 -> ROOut2/1
  MinMax/1 -> Out1/1
  Constant1/1 -> MinMax/1
  Constant3/1 -> MinMax/3

== system c00001M_harness/Eval88 ==
  In2 : Inport
  Constant1 : Constant
  Constant3 : Constant
  Data Type Conversion1 : DataTypeConversion
  Memory2 : Memory  InitialCondition=1
  MinMax : MinMax  Inputs=3
  MinMax2 : MinMax  Inputs=2
  ROOut2 : RelationalOperator  Operator===  OutDataTypeStr=boolean  RndMeth=Simplest
  Out1 : Outport
  wires:
  Data Type Conversion1/1 -> MinMax2/1
  MinMax2/1 -> MinMax/2, Memory2/1
  Memory2/1 -> MinMax2/2
  ROOut2/1 -> Data Type Conversion1/1
  [out2] -> ROOut2/2
  In2/1 -> ROOut2/1
  MinMax/1 -> Out1/1
  Constant1/1 -> MinMax/1
  Constant3/1 -> MinMax/3

== system c00001M_harness/Eval89 ==
  In2 : Inport
  Constant1 : Constant
  Constant3 : Constant
  Data Type Conversion1 : DataTypeConversion
  Memory2 : Memory  InitialCondition=1
  MinMax : MinMax  Inputs=3
  MinMax2 : MinMax  Inputs=2
  ROOut2 : RelationalOperator  Operator===  OutDataTypeStr=boolean  RndMeth=Simplest
  Out1 : Outport
  wires:
  Data Type Conversion1/1 -> MinMax2/1
  MinMax2/1 -> MinMax/2, Memory2/1
  Memory2/1 -> MinMax2/2
  ROOut2/1 -> Data Type Conversion1/1
  [out2] -> ROOut2/2
  In2/1 -> ROOut2/1
  MinMax/1 -> Out1/1
  Constant1/1 -> MinMax/1
  Constant3/1 -> MinMax/3

== system c00001M_harness/Eval90 ==
  In2 : Inport
  Constant1 : Constant
  Constant3 : Constant
  Data Type Conversion1 : DataTypeConversion
  Memory2 : Memory  InitialCondition=1
  MinMax : MinMax  Inputs=3
  MinMax2 : MinMax  Inputs=2
  ROOut2 : RelationalOperator  Operator===  OutDataTypeStr=boolean  RndMeth=Simplest
  Out1 : Outport
  wires:
  Data Type Conversion1/1 -> MinMax2/1
  MinMax2/1 -> MinMax/2, Memory2/1
  Memory2/1 -> MinMax2/2
  ROOut2/1 -> Data Type Conversion1/1
  [out2] -> ROOut2/2
  In2/1 -> ROOut2/1
  MinMax/1 -> Out1/1
  Constant1/1 -> MinMax/1
  Constant3/1 -> MinMax/3

== system c00001M_harness/Eval91 ==
  In2 : Inport
  Constant1 : Constant
  Constant3 : Constant
  Data Type Conversion1 : DataTypeConversion
  Memory2 : Memory  InitialCondition=1
  MinMax : MinMax  Inputs=3
  MinMax2 : MinMax  Inputs=2
  ROOut2 : RelationalOperator  Operator===  OutDataTypeStr=boolean  RndMeth=Simplest
  Out1 : Outport
  wires:
  Data Type Conversion1/1 -> MinMax2/1
  MinMax2/1 -> MinMax/2, Memory2/1
  Memory2/1 -> MinMax2/2
  ROOut2/1 -> Data Type Conversion1/1
  [out2] -> ROOut2/2
  In2/1 -> ROOut2/1
  MinMax/1 -> Out1/1
  Constant1/1 -> MinMax/1
  Constant3/1 -> MinMax/3

== system c00001M_harness/Eval92 ==
  In2 : Inport
  Constant1 : Constant
  Constant3 : Constant
  Data Type Conversion1 : DataTypeConversion
  Memory2 : Memory  InitialCondition=1
  MinMax : MinMax  Inputs=3
  MinMax2 : MinMax  Inputs=2
  ROOut2 : RelationalOperator  Operator===  OutDataTypeStr=boolean  RndMeth=Simplest
  Out1 : Outport
  wires:
  Data Type Conversion1/1 -> MinMax2/1
  MinMax2/1 -> MinMax/2, Memory2/1
  Memory2/1 -> MinMax2/2
  ROOut2/1 -> Data Type Conversion1/1
  [out2] -> ROOut2/2
  In2/1 -> ROOut2/1
  MinMax/1 -> Out1/1
  Constant1/1 -> MinMax/1
  Constant3/1 -> MinMax/3

== system c00001M_harness/Eval93 ==
  In2 : Inport
  Constant1 : Constant
  Constant3 : Constant
  Data Type Conversion1 : DataTypeConversion
  Memory2 : Memory  InitialCondition=1
  MinMax : MinMax  Inputs=3
  MinMax2 : MinMax  Inputs=2
  ROOut2 : RelationalOperator  Operator===  OutDataTypeStr=boolean  RndMeth=Simplest
  Out1 : Outport
  wires:
  Data Type Conversion1/1 -> MinMax2/1
  MinMax2/1 -> MinMax/2, Memory2/1
  Memory2/1 -> MinMax2/2
  ROOut2/1 -> Data Type Conversion1/1
  [out2] -> ROOut2/2
  In2/1 -> ROOut2/1
  MinMax/1 -> Out1/1
  Constant1/1 -> MinMax/1
  Constant3/1 -> MinMax/3

== system c00001M_harness/Eval94 ==
  In2 : Inport
  Constant1 : Constant
  Constant3 : Constant
  Data Type Conversion1 : DataTypeConversion
  Memory2 : Memory  InitialCondition=1
  MinMax : MinMax  Inputs=3
  MinMax2 : MinMax  Inputs=2
  ROOut2 : RelationalOperator  Operator===  OutDataTypeStr=boolean  RndMeth=Simplest
  Out1 : Outport
  wires:
  Data Type Conversion1/1 -> MinMax2/1
  MinMax2/1 -> MinMax/2, Memory2/1
  Memory2/1 -> MinMax2/2
  ROOut2/1 -> Data Type Conversion1/1
  [out2] -> ROOut2/2
  In2/1 -> ROOut2/1
  MinMax/1 -> Out1/1
  Constant1/1 -> MinMax/1
  Constant3/1 -> MinMax/3

== system c00001M_harness/Eval95 ==
  In2 : Inport
  Constant1 : Constant
  Constant3 : Constant
  Data Type Conversion1 : DataTypeConversion
  Memory2 : Memory  InitialCondition=1
  MinMax : MinMax  Inputs=3
  MinMax2 : MinMax  Inputs=2
  ROOut2 : RelationalOperator  Operator===  OutDataTypeStr=boolean  RndMeth=Simplest
  Out1 : Outport
  wires:
  Data Type Conversion1/1 -> MinMax2/1
  MinMax2/1 -> MinMax/2, Memory2/1
  Memory2/1 -> MinMax2/2
  ROOut2/1 -> Data Type Conversion1/1
  [out2] -> ROOut2/2
  In2/1 -> ROOut2/1
  MinMax/1 -> Out1/1
  Constant1/1 -> MinMax/1
  Constant3/1 -> MinMax/3

== system c00001M_harness/Eval96 ==
  In2 : Inport
  Constant1 : Constant
  Constant3 : Constant
  Data Type Conversion1 : DataTypeConversion
  Memory2 : Memory  InitialCondition=1
  MinMax : MinMax  Inputs=3
  MinMax2 : MinMax  Inputs=2
  ROOut2 : RelationalOperator  Operator===  OutDataTypeStr=boolean  RndMeth=Simplest
  Out1 : Outport
  wires:
  Data Type Conversion1/1 -> MinMax2/1
  MinMax2/1 -> MinMax/2, Memory2/1
  Memory2/1 -> MinMax2/2
  ROOut2/1 -> Data Type Conversion1/1
  [out2] -> ROOut2/2
  In2/1 -> ROOut2/1
  MinMax/1 -> Out1/1
  Constant1/1 -> MinMax/1
  Constant3/1 -> MinMax/3

== system c00001M_harness/Eval97 ==
  In2 : Inport
  Constant1 : Constant
  Constant3 : Constant
  Data Type Conversion1 : DataTypeConversion
  Memory2 : Memory  InitialCondition=1
  MinMax : MinMax  Inputs=3
  MinMax2 : MinMax  Inputs=2
  ROOut2 : RelationalOperator  Operator===  OutDataTypeStr=boolean  RndMeth=Simplest
  Out1 : Outport
  wires:
  Data Type Conversion1/1 -> MinMax2/1
  MinMax2/1 -> MinMax/2, Memory2/1
  Memory2/1 -> MinMax2/2
  ROOut2/1 -> Data Type Conversion1/1
  [out2] -> ROOut2/2
  In2/1 -> ROOut2/1
  MinMax/1 -> Out1/1
  Constant1/1 -> MinMax/1
  Constant3/1 -> MinMax/3

== system c00001M_harness/Eval98 ==
  In2 : Inport
  Constant1 : Constant
  Constant3 : Constant
  Data Type Conversion1 : DataTypeConversion
  Memory2 : Memory  InitialCondition=1
  MinMax : MinMax  Inputs=3
  MinMax2 : MinMax  Inputs=2
  ROOut2 : RelationalOperator  Operator===  OutDataTypeStr=boolean  RndMeth=Simplest
  Out1 : Outport
  wires:
  Data Type Conversion1/1 -> MinMax2/1
  MinMax2/1 -> MinMax/2, Memory2/1
  Memory2/1 -> MinMax2/2
  ROOut2/1 -> Data Type Conversion1/1
  [out2] -> ROOut2/2
  In2/1 -> ROOut2/1
  MinMax/1 -> Out1/1
  Constant1/1 -> MinMax/1
  Constant3/1 -> MinMax/3

== system c00001M_harness/Eval99 ==
  In2 : Inport
  Constant1 : Constant
  Constant3 : Constant
  Data Type Conversion1 : DataTypeConversion
  Memory2 : Memory  InitialCondition=1
  MinMax : MinMax  Inputs=3
  MinMax2 : MinMax  Inputs=2
  ROOut2 : RelationalOperator  Operator===  OutDataTypeStr=boolean  RndMeth=Simplest
  Out1 : Outport
  wires:
  Data Type Conversion1/1 -> MinMax2/1
  MinMax2/1 -> MinMax/2, Memory2/1
  Memory2/1 -> MinMax2/2
  ROOut2/1 -> Data Type Conversion1/1
  [out2] -> ROOut2/2
  In2/1 -> ROOut2/1
  MinMax/1 -> Out1/1
  Constant1/1 -> MinMax/1
  Constant3/1 -> MinMax/3

== system c00001M_harness/Inputs ==
  Demux : Demux  Tag=STV Demux  Outputs=3
  FromWs : FromWorkspace  Tag=STV FromWs  VariableName=tuvar  SampleTime=0
  CT2 : Outport  Tag=STV Outport
  T2 : Outport  Tag=STV Outport  Port=2
  EB2 : Outport  Tag=STV Outport  Port=3
  wires:
  Demux/3 -> EB2/1
  Demux/2 -> T2/1
  Demux/1 -> CT2/1
  FromWs/1 -> Demux/1

== system c00001M_harness/M083 ==
  note: VALUES
      | ---------------------------------
      | ControlType = 1 | 2 | 3
      | FillTank = 0 | 1
      | EmptyTank = 0 | 1
      | ManualReference between 0 and 1
      | Tempreature between 0 and 100
      | EmergencyButton = 0 | 1
      | LiquidLevel between 0 and 1 (hmax)
  note: Inputs For Tank2
  note: NAMES
      | --------------------------------------------
      | CT1 = ControlType Tank 1
      | F1 = Fill Tank 1
      | E1 = Empty Tank 1
      | MR1 = Manual Reference Tank1
      | T1 = Temperature Tank 1
      | EB1 = Emergency Button Tank 1
      | LL1 = Liquid Level 1
  note: Inputs For Tank3
  note: Inputs For Tank1
  CT2 : Inport
  T2 : Inport  Port=2
  EB2 : Inport  Port=3
  Tank2 : Subsystem
  LL2 : Outport
  wires:
  Tank2/1(LL2) -> LL2/1
  EB2/1 -> Tank2/3(EB2)
  CT2/1 -> Tank2/1(CT2)
  T2/1 -> Tank2/2(T2)
